simulink model "NewModel"  (R2020a)
settings: Solver=VariableStepAuto  StartTime=0.0  StopTime=500  RelTol=1e-3
values from neighbouring files (symbols this model uses):
  Ctr = 1.6    [ACC_DATA.m]
  F_aero = 1/(2*m_Follower)*Ro_A_Cd    (= 0.00026)    [ACC_DATA.m]
  F_grav = g*sin(theta)    [ACC_DATA.m]
  F_res = g*Cr*cos(theta)    [ACC_DATA.m]
  Kb = 0.08    [ACC_DATA.m]
  Kc = 1    [ACC_DATA.m]
  m_Follower = 1500    [ACC_DATA.m]
  r = 0.326    [ACC_DATA.m]
  Rf = 3.28    [ACC_DATA.m]
  Rtr = 1    [ACC_DATA.m]
  t_gap = 1.4    [ACC_DATA.m]    (also in Untitled.m)
  Tmax = 528.7 + 0.152*Ne - 0.0000217*Ne^2    (= 789.5)    [ACC_DATA.m]
  Ts = 0.1    [ACC_DATA.m]
  v0_lead = 20    [ACC_DATA.m]
  v_set = 40    [ACC_DATA.m]    (also in Untitled.m = 30)
  x0_ego = 10    [ACC_DATA.m]
  x0_lead = 500    [ACC_DATA.m]
undefined symbols (not defined in the file or in its folder): sigbuilder_block
libraries: simulink x2
settings Model: Creator=91968  LastModifiedBy=91968

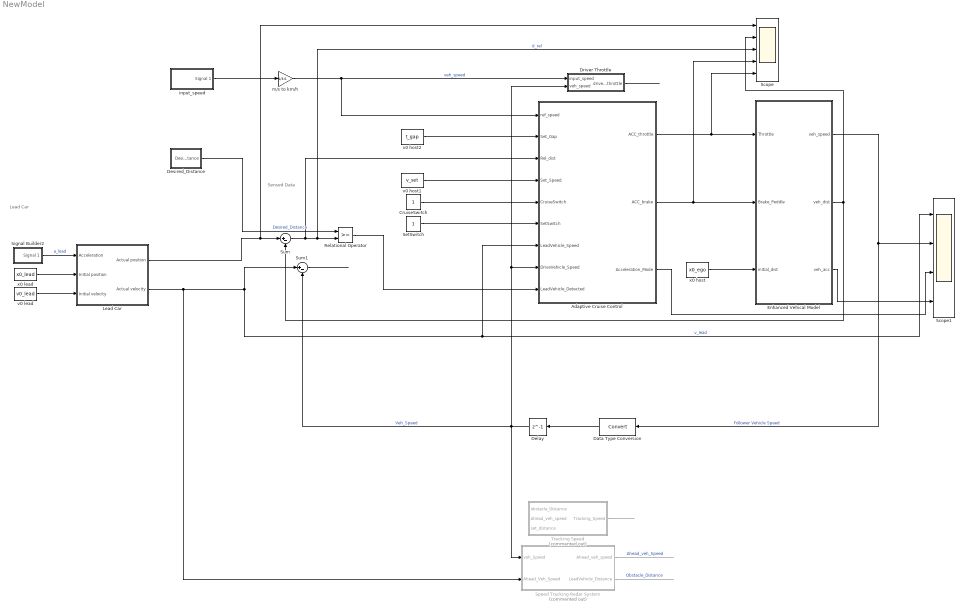
== system NewModel ==
  note: Lead Car
  note: Sensed Data
  Adaptive Cruise Control : Subsystem
  CruiseSwitch : Constant
  Data Type Conversion : DataTypeConversion
  Delay : Delay  DelayLength=1  InitialCondition=0
  Desired_Distance : Subsystem  mask{Desired_Distance=50.0}
      mask DialogControl DescGroupVar Prompt: Set Desired Distance
      mask Display: image('C:\Users\Talha Rao\Pictures\070558928_iconm (2).jpeg');
  Driver Throttle : Subsystem
  Enhanced Vehical Model : Subsystem
  Lead Car : Subsystem
  Relational Operator : RelationalOperator  OutDataTypeStr=boolean  RndMeth=Simplest
  Scope : Scope  NumInputPorts=5
  Scope1 : Scope  NumInputPorts=4
  SetSwitch : Constant
  Signal Builder2 : Subsystem  Tag=STV Subsys  LoadFcn=sigbuilder_block('load');  StartFcn=sigbuilder_block('start');  StopFcn=sigbuilder_block('stop');  ClipboardFcn=sigbuilder_block('clipboard');  mask(Sigbuilder block){tuvar=[0:10]}
      mask help: Simulink:masks:SigbuilderBlock_MD
      mask init:
      | if ~strcmp(get_param(bdroot(gcbh),'SimulationStatus'),'stopped') tuvar = sigbuilder_block('maskInit'); end
      settings: CopyFcn=sigbuilder_block('copy');  DeleteFcn=sigbuilder_block('delete');  ModelCloseFcn=sigbuilder_block('modelClose');  PreSaveFcn=sigbuilder_block('preSave');  PauseFcn=sigbuilder_block('pause');  ContinueFcn=sigbuilder_block('continue');  NameChangeFcn=sigbuilder_block('namechange');  OpenFcn=sigbuilder_block('open',[883.5 285.75 550.5 318.75 ]);  CloseFcn=sigbuilder_block('close');
      mask Display: plot(0, 0, 100, 100,[2, 2, 32, 32, 2], [68, 8, 8, 68, 68],[32, 2], [38, 38], [32, 19, 2],[53, 60, 44], [32, 17, 17, 2],[16, 16, 31, 31]);txt = getActiveGroup(gcbh);text(2, 100, txt,'verticalAlignment', 'top');
  Speed Tracking Redar System : Subsystem  Commented=on
  Sum : Sum  Inputs=|+-
  Sum1 : Sum  Inputs=|+-
  Tracking Speed : Subsystem  Commented=on
  input_speed : Subsystem  Tag=STV Subsys  LoadFcn=sigbuilder_block('load');  StartFcn=sigbuilder_block('start');  StopFcn=sigbuilder_block('stop');  ClipboardFcn=sigbuilder_block('clipboard');  mask(Sigbuilder block){tuvar=[0:10]}
      mask help: Simulink:masks:SigbuilderBlock_MD
      mask init:
      | if ~strcmp(get_param(bdroot(gcbh),'SimulationStatus'),'stopped') tuvar = sigbuilder_block('maskInit'); end
      settings: CopyFcn=sigbuilder_block('copy');  DeleteFcn=sigbuilder_block('delete');  ModelCloseFcn=sigbuilder_block('modelClose');  PreSaveFcn=sigbuilder_block('preSave');  PauseFcn=sigbuilder_block('pause');  ContinueFcn=sigbuilder_block('continue');  NameChangeFcn=sigbuilder_block('namechange');  OpenFcn=sigbuilder_block('open',[167.25 146.25 1152 549.75 ]);  CloseFcn=sigbuilder_block('close');
      mask Display: plot(0, 0, 100, 100,[2, 2, 32, 32, 2], [68, 8, 8, 68, 68],[32, 2], [38, 38], [32, 19, 2],[53, 60, 44], [32, 17, 17, 2],[16, 16, 31, 31]);txt = getActiveGroup(gcbh);text(2, 100, txt,'verticalAlignment', 'top');
  m/s to km/h : Gain  Gain=1/3.6
  v0 host1 : Constant  Value=v_set  SampleTime=Ts
  v0 host2 : Constant  Value=t_gap  SampleTime=Ts
  v0 lead : Constant  Value=v0_lead  SampleTime=Ts
  x0 host : Constant  Value=x0_ego  SampleTime=Ts
  x0 lead : Constant  Value=x0_lead  SampleTime=Ts
  wires:
  x0 lead/1 -> Lead Car/2(Initial position)
  v0 lead/1 -> Lead Car/3(Initial velocity)
  Signal Builder2/1(Signal 1) -> Lead Car/1(Acceleration)  "a_lead"
  Lead Car/1(Actual position) -> Scope/1, Sum/1
  Lead Car/2(Actual velocity) -> Speed Tracking Redar System/2(Ahead_Veh_Speed), Scope1/1, Adaptive Cruise Control/7(LeadVehicle_Speed), Sum1/1  "v_lead"
  Delay/1 -> Speed Tracking Redar System/1(veh_Speed), Sum1/2, Adaptive Cruise Control/8(DriveVehicle_Speed), Driver Throttle/2(veh_speed)  "Veh_Speed"
  Speed Tracking Redar System/2(LeadVehicle_Distance) -> ?  "Obstacle_Distance"
  Speed Tracking Redar System/1(Ahead_veh_speed) -> ?  "Ahead_veh_Speed"
  Desired_Distance/1(Desired_Distance) -> Relational Operator/1  "Desired_Distance"
  Enhanced Vehical Model/1(veh_speed) -> Scope1/2, Data Type Conversion/1  "Follower Vehicle Speed"
  Sum/1 -> Scope/3, Relational Operator/2, Adaptive Cruise Control/3(Rel_dist)  "d_rel"
  x0 host/1 -> Enhanced Vehical Model/3(initial_dist)
  Enhanced Vehical Model/2(veh_dist) -> Sum/2, Scope/2
  Data Type Conversion/1 -> Delay/1
  v0 host2/1 -> Adaptive Cruise Control/2(Set_Gap)
  v0 host1/1 -> Adaptive Cruise Control/4(Set_Speed)
  CruiseSwitch/1 -> Adaptive Cruise Control/5(CruiseSwitch)
  SetSwitch/1 -> Adaptive Cruise Control/6(SetSwitch)
  Relational Operator/1 -> Adaptive Cruise Control/9(LeadVehicle_Detected)
  input_speed/1(Signal 1) -> m/s to km/h/1
  Adaptive Cruise Control/1(ACC_throttle) -> Scope/5, Enhanced Vehical Model/1(Throttle)
  Adaptive Cruise Control/2(ACC_brake) -> Scope/4, Enhanced Vehical Model/2(Brake_Peddle)
  Tracking Speed/1(Tracking_Speed) -> ?
  Sum1/1 -> ?
  Driver Throttle/1(driver_throttle) -> ?
  Enhanced Vehical Model/3(veh_acc) -> Scope1/4
  Adaptive Cruise Control/3(Acceleration_Mode) -> Scope1/3
  m/s to km/h/1 -> Adaptive Cruise Control/1(ref_speed), Driver Throttle/1(input_speed)  "veh_speed"

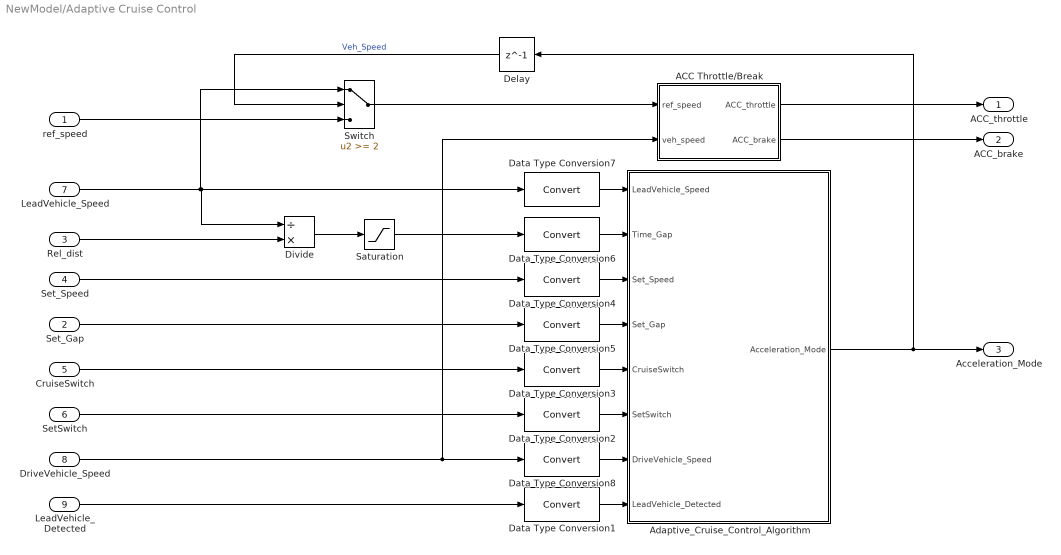
== system NewModel/Adaptive Cruise Control ==
  ref_speed : Inport
  Set_Gap : Inport  Port=2
  Rel_dist : Inport  Port=3
  Set_Speed : Inport  Port=4
  CruiseSwitch : Inport  Port=5
  SetSwitch : Inport  Port=6
  LeadVehicle_Speed : Inport  Port=7  OutMin=0  OutMax=255
  DriveVehicle_Speed : Inport  Port=8  OutMin=0  OutMax=255
  LeadVehicle_Detected : Inport  Port=9  OutMin=0  OutMax=1
  ACC Throttle/Break : Subsystem
  Adaptive_Cruise_Control_Algorithm : Subsystem
  Data Type Conversion{1..8} (8 alike) : DataTypeConversion
  Delay : Delay  DelayLength=1  InitialCondition=0
  Divide : Product  Inputs=/*
  Saturation : Saturate  UpperLimit=100  LowerLimit=0
  Switch : Switch  Threshold=2  SaturateOnIntegerOverflow=on  InputSameDT=on
  ACC_throttle : Outport
  ACC_brake : Outport  Port=2
  Acceleration_Mode : Outport  Port=3
  wires:
  Data Type Conversion7/1 -> Adaptive_Cruise_Control_Algorithm/1(LeadVehicle_Speed)
  Data Type Conversion4/1 -> Adaptive_Cruise_Control_Algorithm/3(Set_Speed)
  Data Type Conversion2/1 -> Adaptive_Cruise_Control_Algorithm/6(SetSwitch)
  Set_Speed/1 -> Data Type Conversion4/1
  Adaptive_Cruise_Control_Algorithm/1(Acceleration_Mode) -> Delay/1, Acceleration_Mode/1
  Data Type Conversion8/1 -> Adaptive_Cruise_Control_Algorithm/7(DriveVehicle_Speed)
  Data Type Conversion6/1 -> Adaptive_Cruise_Control_Algorithm/2(Time_Gap)
  Data Type Conversion3/1 -> Adaptive_Cruise_Control_Algorithm/5(CruiseSwitch)
  Data Type Conversion5/1 -> Adaptive_Cruise_Control_Algorithm/4(Set_Gap)
  Data Type Conversion1/1 -> Adaptive_Cruise_Control_Algorithm/8(LeadVehicle_Detected)
  Set_Gap/1 -> Data Type Conversion5/1
  Divide/1 -> Saturation/1
  ACC Throttle/Break/1(ACC_throttle) -> ACC_throttle/1
  CruiseSwitch/1 -> Data Type Conversion3/1
  ACC Throttle/Break/2(ACC_brake) -> ACC_brake/1
  LeadVehicle_Detected/1 -> Data Type Conversion1/1
  SetSwitch/1 -> Data Type Conversion2/1
  ref_speed/1 -> Switch/3
  DriveVehicle_Speed/1 -> ACC Throttle/Break/2(veh_speed), Data Type Conversion8/1
  LeadVehicle_Speed/1 -> Divide/1, Data Type Conversion7/1, Switch/1
  Rel_dist/1 -> Divide/2
  Saturation/1 -> Data Type Conversion6/1
  Switch/1 -> ACC Throttle/Break/1(ref_speed)
  Delay/1 -> Switch/2  "Veh_Speed"

== system NewModel/Desired_Distance ==
  Constant : Constant  Value=Desired_Distance
  Desired_Distance : Outport  VectorParamsAs1DForOutWhenUnconnected=off
  wires:
  Constant/1 -> Desired_Distance/1

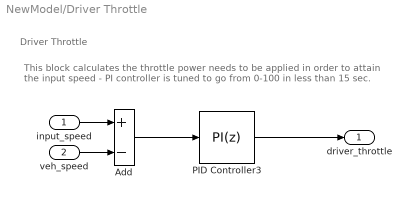
== system NewModel/Driver Throttle ==
  note: This block calculates the throttle power needs to be applied in order to attain the input speed
      | - PI controller is tuned to go from 0-100 in less than 15 sec.
  note: Driver Throttle
  input_speed : Inport
  veh_speed : Inport  Port=2
  Add : Sum  Inputs=+-
  PID Controller3 : simulink/Continuous/PID Controller  Controller=PI  Form=Parallel  TimeDomain=Discrete-time  UseExternalTs=off  SampleTime=0.02  IntegratorMethod=Trapezoidal  FilterMethod=Forward Euler  ControllerParametersSource=internal  P=5  I=0.5  D=0  UseFilter=on  N=100  TunerSelectOption=Transfer Function Based (PID Tuner App)  InitialConditionSource=internal  InitialConditionForIntegrator=0  InitialConditionForFilter=0  DifferentiatorICPrevScaledInput=0  ExternalReset=none  TrackingMode=off  Kt=1  LimitOutput=on  UpperSaturationLimit=100  LowerSaturationLimit=-100  LinearizeAsGain=on  AntiWindupMode=clamping  Kb=1  POutMin=[]  POutMax=[]  IOutMin=[]  IOutMax=[]  DOutMin=[]  DOutMax=[]  NOutMin=[]  NOutMax=[]  SumOutMin=[]  SumOutMax=[]  SaturationOutMin=[]  SaturationOutMax=[]  PParamMin=[]  PParamMax=[]  IParamMin=[]  IParamMax=[]  DParamMin=[]  DParamMax=[]  NParamMin=[]  NParamMax=[]  KbParamMin=[]  KbParamMax=[]  KtParamMin=[]  KtParamMax=[]  KbOutMin=[]  KbOutMax=[]  KtOutMin=[]  KtOutMax=[]  IntegratorOutMin=[]  IntegratorOutMax=[]  FilterOutMin=[]  FilterOutMax=[]  SumI1OutMin=[]  SumI1OutMax=[]  SumI2OutMin=[]  SumI2OutMax=[]  SumI3OutMin=[]  SumI3OutMax=[]  SumI4OutMin=[]  SumI4OutMax=[]  SumDOutMin=[]  SumDOutMax=[]  DifferentiatorOutMin=[]  DifferentiatorOutMax=[]  FilterDiffOutCoefMin=[]  FilterDiffOutCoefMax=[]  ReciprocalOutMin=[]  ReciprocalOutMax=[]  SumDenOutMin=[]  SumDenOutMax=[]  SumNumOutMin=[]  SumNumOutMax=[]  DivideOutMin=[]  DivideOutMax=[]  UdiffTsProdOutMin=[]  UdiffTsProdOutMax=[]  NTsProdOutMin=[]  NTsProdOutMax=[]  UintegralTsProdOutMin=[]  UintegralTsProdOutMax=[]  UngainTsProdOutMin=[]  UngainTsProdOutMax=[]  IntegratorContinuousStateAttributes=''  IntegratorStateMustResolveToSignalObject=off  IntegratorRTWStateStorageClass=Auto  FilterContinuousStateAttributes=''  FilterStateMustResolveToSignalObject=off  FilterRTWStateStorageClass=Auto  ParallelPVariant=InternalParameters  IdealPVariant=Disabled  IVariant=InternalParameters  DVariant=Disabled  IntegratorVariant=Discrete  SatVariant=Enabled  AWVariant=DiscClampingParallel  PCopyVariant=Disabled  TRVariant=Disabled  FdbkBlocksVariant=Feedback  IdealPFdbkVariant=Passthrough  SatFdbkVariant=Passthrough  DerivativeFilterVariant=Disabled  NVariant=Disabled  NCopyVariant=Disabled_SignalSpec  FilterICVariant=Disabled  IntegratorICVariant=InternalICs  ExternalResetVariant=Disabled  TRSumVariant=Passthrough  SumFdbkVariant=Enabled  SumVariant=Sum_PI  TsampFilterVariant=InternalTs  TsampNgainVariant=Passthrough  TsampIntegralVariant=Passthrough
  driver_throttle : Outport  VectorParamsAs1DForOutWhenUnconnected=off
  wires:
  input_speed/1 -> Add/1
  veh_speed/1 -> Add/2
  PID Controller3/1 -> driver_throttle/1
  Add/1 -> PID Controller3/1

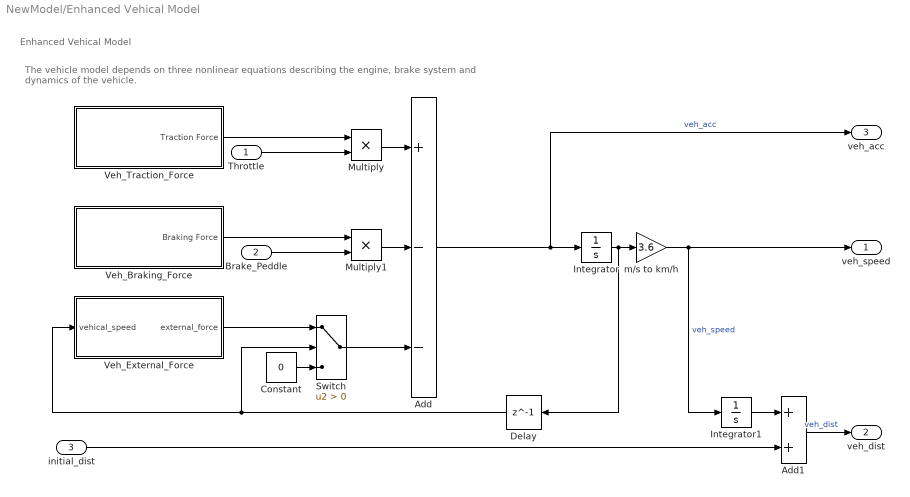
== system NewModel/Enhanced Vehical Model ==
  note: The vehicle model depends on three nonlinear equations describing the engine, brake system and dynamics of the vehicle.
  note: Enhanced Vehical Model
  Throttle : Inport
  Brake_Peddle : Inport  Port=2
  initial_dist : Inport  Port=3
  Add : Sum  Inputs=+--
  Add1 : Sum
  Constant : Constant  Value=0
  Delay : Delay  DelayLength=1  InitialCondition=0
  Integrator : Integrator
  Integrator1 : Integrator
  Multiply : Product
  Multiply1 : Product
  Switch : Switch  Criteria=u2 > Threshold  SaturateOnIntegerOverflow=on  InputSameDT=on
  Veh_Braking_Force : Subsystem
  Veh_External_Force : Subsystem
  Veh_Traction_Force : Subsystem
  m/s to km/h : Gain  Gain=3.6
  veh_speed : Outport  VectorParamsAs1DForOutWhenUnconnected=off
  veh_dist : Outport  Port=2  VectorParamsAs1DForOutWhenUnconnected=off
  veh_acc : Outport  Port=3  VectorParamsAs1DForOutWhenUnconnected=off
  wires:
  Switch/1 -> Add/3
  Brake_Peddle/1 -> Multiply1/2
  Veh_Braking_Force/1("Braking Force ") -> Multiply1/1
  Multiply1/1 -> Add/2
  Multiply/1 -> Add/1
  Veh_Traction_Force/1(Traction Force) -> Multiply/1
  Integrator/1 -> Delay/1, m/s to km/h/1
  m/s to km/h/1 -> Integrator1/1, veh_speed/1  "veh_speed"
  Integrator1/1 -> Add1/1
  Add1/1 -> veh_dist/1  "veh_dist"
  initial_dist/1 -> Add1/2
  Delay/1 -> Switch/2, Veh_External_Force/1(vehical_speed)
  Veh_External_Force/1(external_force) -> Switch/1
  Constant/1 -> Switch/3
  Add/1 -> veh_acc/1, Integrator/1  "veh_acc"
  Throttle/1 -> Multiply/2

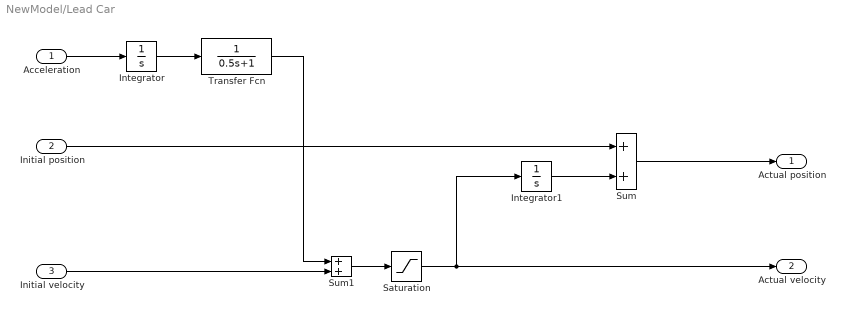
== system NewModel/Lead Car ==
  Acceleration : Inport
  Initial position : Inport  Port=2
  Initial velocity : Inport  Port=3
  Integrator : Integrator
  Integrator1 : Integrator
  Saturation : Saturate  UpperLimit=50  LowerLimit=0
  Sum : Sum
  Sum1 : Sum
  Transfer Fcn : TransferFcn  Denominator=[0.5 1]
  Actual position : Outport  VectorParamsAs1DForOutWhenUnconnected=off
  Actual velocity : Outport  Port=2  VectorParamsAs1DForOutWhenUnconnected=off
  wires:
  Transfer Fcn/1 -> Sum1/1
  Initial velocity/1 -> Sum1/2
  Sum/1 -> Actual position/1
  Integrator/1 -> Transfer Fcn/1
  Sum1/1 -> Saturation/1
  Acceleration/1 -> Integrator/1
  Initial position/1 -> Sum/1
  Integrator1/1 -> Sum/2
  Saturation/1 -> Integrator1/1, Actual velocity/1

== system NewModel/Signal Builder2 ==
  Demux : Demux  Tag=STV Demux  Outputs=1
      settings: DisplayOption=none
  FromWs : FromWorkspace  Tag=STV FromWs  VariableName=tuvar
      SigBuilderData=|
      | common.afterFinalStr = 'Extrapolate'
      | common.sampleTime = 0
      | dataSet.timeRange = [0 500]
      | dataSet.name = 'Group 1'
      | sbobj.Groups.Name = 'Group 1'
      | sbobj.Groups.Signals.Name = 'Signal 1'
      | sbobj.Groups.Signals.XData = [0 20 30 40 60 80 100 150 200 250 300 350 400 451 500]
      | sbobj.Groups.Signals.YData = [0.5 1 1.5 1.5 0.75 -1 -1.8 0 -0.5 -3 0.5 -0.25 -1 -1 -1.5]
      | sbobj.Groups.TimeRange = [0 500]
  Signal 1 : Outport  Tag=STV Outport
  wires:
  Demux/1 -> Signal 1/1
  FromWs/1 -> Demux/1

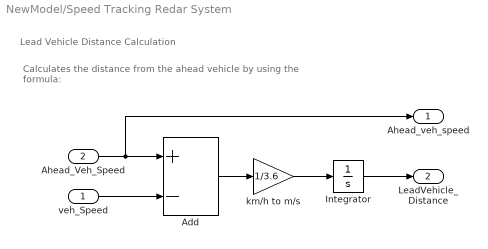
== system NewModel/Speed Tracking Redar System ==
  note: Calculates the distance from the ahead vehicle by using the formula:
  note: Lead Vehicle Distance Calculation
  veh_Speed : Inport
  Ahead_Veh_Speed : Inport  Port=2
  Add : Sum  Inputs=+-
  Integrator : Integrator  InitialCondition=100
  km/h to m/s : Gain  Gain=1/3.6
  Ahead_veh_speed : Outport  VectorParamsAs1DForOutWhenUnconnected=off
  LeadVehicle_Distance : Outport  Port=2  VectorParamsAs1DForOutWhenUnconnected=off
  wires:
  Ahead_Veh_Speed/1 -> Ahead_veh_speed/1, Add/1
  veh_Speed/1 -> Add/2
  Add/1 -> km/h to m/s/1
  km/h to m/s/1 -> Integrator/1
  Integrator/1 -> LeadVehicle_Distance/1

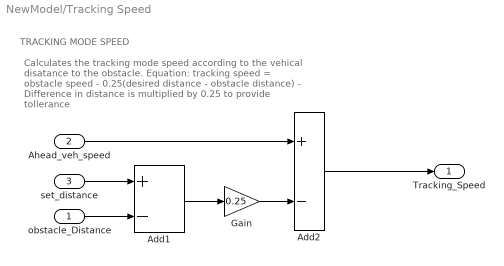
== system NewModel/Tracking Speed ==
  note: Calculates the tracking mode speed according to the vehical disatance
      | to the obstacle.
      | Equation:
      |
      | tracking speed = obstacle speed - 0.25(desired distance - obstacle distance)
      |
      | - Difference in distance is multiplied by 0.25 to provide tollerance
  note: TRACKING MODE SPEED
  obstacle_Distance : Inport
  Ahead_veh_speed : Inport  Port=2
  set_distance : Inport  Port=3
  Add1 : Sum  Inputs=+-
  Add2 : Sum  Inputs=+-
  Gain : Gain  Gain=0.25
  Tracking_Speed : Outport  VectorParamsAs1DForOutWhenUnconnected=off
  wires:
  Add1/1 -> Gain/1
  Gain/1 -> Add2/2
  Ahead_veh_speed/1 -> Add2/1
  Add2/1 -> Tracking_Speed/1
  set_distance/1 -> Add1/1
  obstacle_Distance/1 -> Add1/2

== system NewModel/input_speed ==
  Demux : Demux  Tag=STV Demux  Outputs=1
      settings: DisplayOption=none
  FromWs : FromWorkspace  Tag=STV FromWs  VariableName=tuvar
      SigBuilderData=|
      | common.afterFinalStr = 'Extrapolate'
      | common.sampleTime = 0
      | dataSet.timeRange = [0 500]
      | dataSet.name = 'Group 1'
      | sbobj.Groups.Name = 'Group 1'
      | sbobj.Groups.Signals.Name = 'Signal 1'
      | sbobj.Groups.Signals.XData = [0 20 30 40 60 80 100 150 200 250 300 350 400 451 500]
      | sbobj.Groups.Signals.YData = [0.5 15.5 25.5 40.5 40.5 75.5 75.5 70.5 60.5 60 90 90 60 45 40]
      | sbobj.Groups.TimeRange = [0 500]
  Signal 1 : Outport  Tag=STV Outport
  wires:
  Demux/1 -> Signal 1/1
  FromWs/1 -> Demux/1

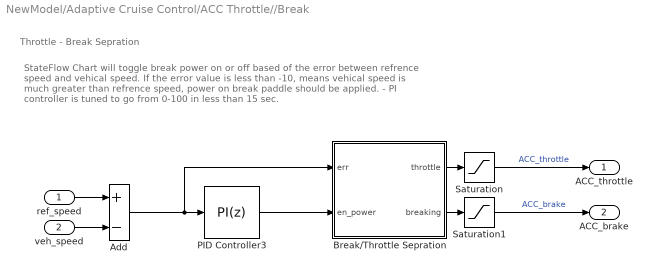
== system NewModel/Adaptive Cruise Control/ACC Throttle//Break ==
  note: StateFlow Chart will toggle break power on or off based of the error between refrence speed and
      | vehical speed. If the error value is less than -10, means vehical speed is much greater than refrence
      | speed, power on break paddle should be applied.
      |
      | - PI controller is tuned to go from 0-100 in less than 15 sec.
  note: Throttle - Break Sepration
  ref_speed : Inport
  veh_speed : Inport  Port=2
  Add : Sum  Inputs=+-
  Break/Throttle Sepration : Stateflow chart  TreatAsAtomicUnit=on
  PID Controller3 : simulink/Continuous/PID Controller  Controller=PI  Form=Parallel  TimeDomain=Discrete-time  UseExternalTs=off  SampleTime=0.02  IntegratorMethod=Trapezoidal  FilterMethod=Forward Euler  ControllerParametersSource=internal  P=2  I=5  D=0  UseFilter=on  N=100  TunerSelectOption=Transfer Function Based (PID Tuner App)  InitialConditionSource=internal  InitialConditionForIntegrator=0  InitialConditionForFilter=0  DifferentiatorICPrevScaledInput=0  ExternalReset=none  TrackingMode=off  Kt=1  LimitOutput=on  UpperSaturationLimit=100  LowerSaturationLimit=-100  LinearizeAsGain=on  AntiWindupMode=clamping  Kb=1  POutMin=[]  POutMax=[]  IOutMin=[]  IOutMax=[]  DOutMin=[]  DOutMax=[]  NOutMin=[]  NOutMax=[]  SumOutMin=[]  SumOutMax=[]  SaturationOutMin=[]  SaturationOutMax=[]  PParamMin=[]  PParamMax=[]  IParamMin=[]  IParamMax=[]  DParamMin=[]  DParamMax=[]  NParamMin=[]  NParamMax=[]  KbParamMin=[]  KbParamMax=[]  KtParamMin=[]  KtParamMax=[]  KbOutMin=[]  KbOutMax=[]  KtOutMin=[]  KtOutMax=[]  IntegratorOutMin=[]  IntegratorOutMax=[]  FilterOutMin=[]  FilterOutMax=[]  SumI1OutMin=[]  SumI1OutMax=[]  SumI2OutMin=[]  SumI2OutMax=[]  SumI3OutMin=[]  SumI3OutMax=[]  SumI4OutMin=[]  SumI4OutMax=[]  SumDOutMin=[]  SumDOutMax=[]  DifferentiatorOutMin=[]  DifferentiatorOutMax=[]  FilterDiffOutCoefMin=[]  FilterDiffOutCoefMax=[]  ReciprocalOutMin=[]  ReciprocalOutMax=[]  SumDenOutMin=[]  SumDenOutMax=[]  SumNumOutMin=[]  SumNumOutMax=[]  DivideOutMin=[]  DivideOutMax=[]  UdiffTsProdOutMin=[]  UdiffTsProdOutMax=[]  NTsProdOutMin=[]  NTsProdOutMax=[]  UintegralTsProdOutMin=[]  UintegralTsProdOutMax=[]  UngainTsProdOutMin=[]  UngainTsProdOutMax=[]  IntegratorContinuousStateAttributes=''  IntegratorStateMustResolveToSignalObject=off  IntegratorRTWStateStorageClass=Auto  FilterContinuousStateAttributes=''  FilterStateMustResolveToSignalObject=off  FilterRTWStateStorageClass=Auto  ParallelPVariant=InternalParameters  IdealPVariant=Disabled  IVariant=InternalParameters  DVariant=Disabled  IntegratorVariant=Discrete  SatVariant=Enabled  AWVariant=DiscClampingParallel  PCopyVariant=Disabled  TRVariant=Disabled  FdbkBlocksVariant=Feedback  IdealPFdbkVariant=Passthrough  SatFdbkVariant=Passthrough  DerivativeFilterVariant=Disabled  NVariant=Disabled  NCopyVariant=Disabled_SignalSpec  FilterICVariant=Disabled  IntegratorICVariant=InternalICs  ExternalResetVariant=Disabled  TRSumVariant=Passthrough  SumFdbkVariant=Enabled  SumVariant=Sum_PI  TsampFilterVariant=InternalTs  TsampNgainVariant=Passthrough  TsampIntegralVariant=Passthrough
  Saturation : Saturate  UpperLimit=50  LowerLimit=0
  Saturation1 : Saturate  UpperLimit=20  LowerLimit=0
  ACC_throttle : Outport  VectorParamsAs1DForOutWhenUnconnected=off
  ACC_brake : Outport  Port=2  VectorParamsAs1DForOutWhenUnconnected=off
  wires:
  ref_speed/1 -> Add/1
  veh_speed/1 -> Add/2
  Break/Throttle Sepration/1(throttle) -> Saturation/1
  Break/Throttle Sepration/2(breaking) -> Saturation1/1
  PID Controller3/1 -> Break/Throttle Sepration/2(en_power)
  Add/1 -> Break/Throttle Sepration/1(err), PID Controller3/1
  Saturation/1 -> ACC_throttle/1  "ACC_throttle"
  Saturation1/1 -> ACC_brake/1  "ACC_brake"

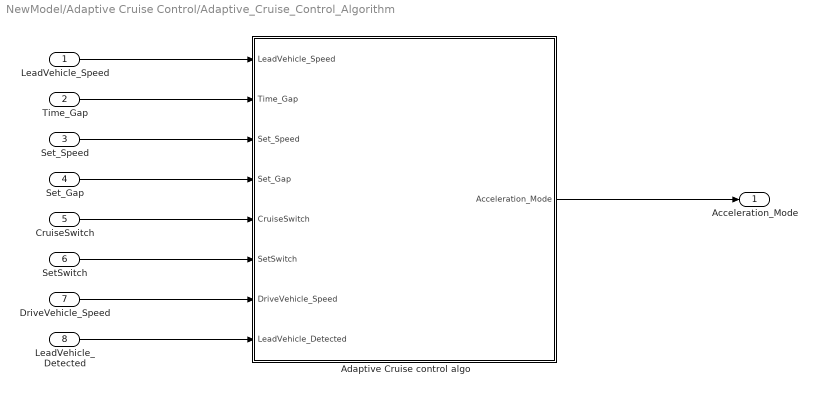
== system NewModel/Adaptive Cruise Control/Adaptive_Cruise_Control_Algorithm ==
  LeadVehicle_Speed : Inport  OutMin=0  OutMax=255
  Time_Gap : Inport  Port=2
  Set_Speed : Inport  Port=3
  Set_Gap : Inport  Port=4
  CruiseSwitch : Inport  Port=5
  SetSwitch : Inport  Port=6
  DriveVehicle_Speed : Inport  Port=7  OutMin=0  OutMax=255
  LeadVehicle_Detected : Inport  Port=8  OutMin=0  OutMax=255
  Adaptive Cruise control algo : Stateflow chart  RequirementInfo={} %GIDa_57645b32_15f0_49df_b2ac_141007f7ec66  TreatAsAtomicUnit=on
  Acceleration_Mode : Outport  OutMin=0  OutMax=255
  wires:
  LeadVehicle_Speed/1 -> Adaptive Cruise control algo/1(LeadVehicle_Speed)
  Set_Gap/1 -> Adaptive Cruise control algo/4(Set_Gap)
  Set_Speed/1 -> Adaptive Cruise control algo/3(Set_Speed)
  Time_Gap/1 -> Adaptive Cruise control algo/2(Time_Gap)
  LeadVehicle_Detected/1 -> Adaptive Cruise control algo/8(LeadVehicle_Detected)
  DriveVehicle_Speed/1 -> Adaptive Cruise control algo/7(DriveVehicle_Speed)
  SetSwitch/1 -> Adaptive Cruise control algo/6(SetSwitch)
  CruiseSwitch/1 -> Adaptive Cruise control algo/5(CruiseSwitch)
  Adaptive Cruise control algo/1(Acceleration_Mode) -> Acceleration_Mode/1

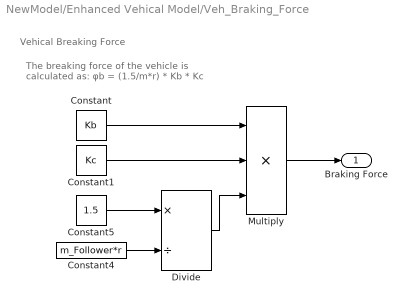
== system NewModel/Enhanced Vehical Model/Veh_Braking_Force ==
  note: Vehical Breaking Force
  note: The breaking force of the vehicle is calculated as:
      | φb = (1.5/m*r) * Kb * Kc
  Constant : Constant  Value=Kb
  Constant1 : Constant  Value=Kc
  Constant4 : Constant  Value=m_Follower*r
  Constant5 : Constant  Value=1.5
  Divide : Product  Inputs=*/
  Multiply : Product  Inputs=3
  "Braking Force " : Outport  VectorParamsAs1DForOutWhenUnconnected=off
  wires:
  Multiply/1 -> "Braking Force "/1
  Constant4/1 -> Divide/2
  Constant1/1 -> Multiply/2
  Constant/1 -> Multiply/1
  Constant5/1 -> Divide/1
  Divide/1 -> Multiply/3

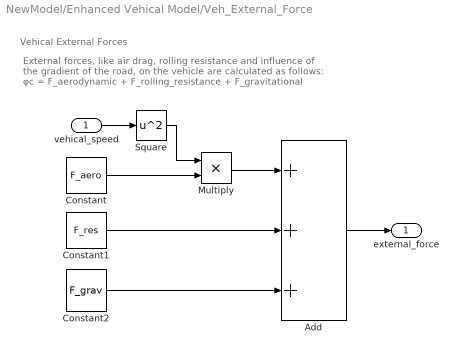
== system NewModel/Enhanced Vehical Model/Veh_External_Force ==
  note: External forces, like air drag, rolling resistance and
      | influence of the gradient of the road, on the vehicle are calculated as follows:
      |
      | φc = F_aerodynamic + F_rolling_resistance + F_gravitational
  note: Vehical External Forces
  vehical_speed : Inport
  Add : Sum  Inputs=+++
  Constant : Constant  Value=F_aero
  Constant1 : Constant  Value=F_res
  Constant2 : Constant  Value=F_grav
  Multiply : Product
  Square : Math  Operator=square  SignedPower=on  SaturateOnIntegerOverflow=on
  external_force : Outport  VectorParamsAs1DForOutWhenUnconnected=off
  wires:
  Add/1 -> external_force/1
  Constant1/1 -> Add/2
  Constant2/1 -> Add/3
  Constant/1 -> Multiply/2
  vehical_speed/1 -> Square/1
  Square/1 -> Multiply/1
  Multiply/1 -> Add/1

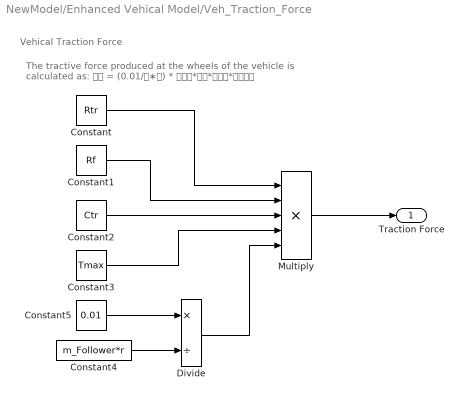
== system NewModel/Enhanced Vehical Model/Veh_Traction_Force ==
  note: The tractive force produced at the wheels of the vehicle is calculated as:
      | 𝜑𝑡 = (0.01/𝑚∗𝑟) * 𝑅𝑡𝑟*𝑅𝑓*𝐶𝑡𝑟*𝑇𝑚𝑎𝑥
  note: Vehical Traction Force
  Constant : Constant  Value=Rtr
  Constant1 : Constant  Value=Rf
  Constant2 : Constant  Value=Ctr
  Constant3 : Constant  Value=Tmax
  Constant4 : Constant  Value=m_Follower*r
  Constant5 : Constant  Value=0.01
  Divide : Product  Inputs=*/
  Multiply : Product  Inputs=5
  Traction Force : Outport  VectorParamsAs1DForOutWhenUnconnected=off
  wires:
  Constant/1 -> Multiply/1
  Constant4/1 -> Divide/2
  Constant1/1 -> Multiply/2
  Constant5/1 -> Divide/1
  Constant3/1 -> Multiply/4
  Divide/1 -> Multiply/5
  Constant2/1 -> Multiply/3
  Multiply/1 -> Traction Force/1

== stateflow chart NewModel/Adaptive Cruise Control/ACC Throttle//Break/Break//Throttle Sepration ==
  note: Break/Throttle Separation
  note: State
      | Description
      | Condition
      | Next State
      |
      | OPEN_THROTTLE
      | Apply power on throttle when error is >= -10
      | err >= -10
      | APPLY_BREAK
      |
      | APPLY_BREAK
      | Apply power on break when error is < -10
      | err < -10
      | OPEN_THROTTLE
  state OPEN_THROTTLE
    en: breaking = 0;
    during: throttle = en_power;
  state APPLY_BREAK
    during: breaking = en_power;
    en:throttle = 0;
  (default) -> OPEN_THROTTLE
  OPEN_THROTTLE -> APPLY_BREAK : [err<-5]
  APPLY_BREAK -> OPEN_THROTTLE : [err >= 0]
  data: throttle output; breaking output; err input; en_power input

== stateflow chart NewModel/Adaptive Cruise Control/Adaptive_Cruise_Control_Algorithm/Adaptive Cruise control algo ==
  state ACC_STANDBY_MODE
    entry:
    Acceleration_Mode = 1;
  state ACC_OFF_MODE
    entry:
    Acceleration_Mode = 0;
  state ACC_ON_MODE
    state LeadVehicle_Not_Detected_Resume
      entry:
      Acceleration_Mode= 1;
    state LeadVehicle_Detected_Resume
      entry:
      Acceleration_Mode= 3;
    state LeadVehicle_Detected_Follow
      entry:
      Acceleration_Mode= 2;
    state LeadVehicle_Not_Detected
      entry:
      Acceleration_Mode= 1;
    state LeadVehicle_Speed_equal_Set_Speed
      entry:
      Acceleration_Mode= 4;
    state LeadVehicle_Speed_lessthan_Set_Speed
      entry:
      Acceleration_Mode= 5;
    (default) -> LeadVehicle_Detected_Follow
    LeadVehicle_Detected_Resume -> LeadVehicle_Not_Detected_Resume [order 1] : [LeadVehicle_Detected ==0]
    LeadVehicle_Detected_Follow -> LeadVehicle_Detected_Resume [order 3] : [(DriveVehicle_Speed==Set_Speed) ...
        | && (LeadVehicle_Speed >= Set_Speed)...
        |  && (Time_Gap>=Set_Gap)]
    LeadVehicle_Speed_lessthan_Set_Speed -> LeadVehicle_Not_Detected_Resume [order 2] : [(LeadVehicle_Detected==0) ...
        | || (DriveVehicle_Speed <= Set_Speed)]
    LeadVehicle_Detected_Resume -> LeadVehicle_Speed_lessthan_Set_Speed [order 2] : [(DriveVehicle_Speed< Set_Speed) ...
        | && (LeadVehicle_Speed > DriveVehicle_Speed)...
        | || (Time_Gap >= Set_Gap)]
    LeadVehicle_Speed_lessthan_Set_Speed -> LeadVehicle_Detected_Resume [order 1] : [(DriveVehicle_Speed< Set_Speed) ...
        | && (LeadVehicle_Speed > DriveVehicle_Speed)...
        | && (Time_Gap >= Set_Gap)]
    LeadVehicle_Detected_Follow -> LeadVehicle_Not_Detected [order 2] : [LeadVehicle_Detected ==0]
    LeadVehicle_Not_Detected -> LeadVehicle_Detected_Follow [order 1] : [(LeadVehicle_Detected==1) && ...
        | (DriveVehicle_Speed == Set_Speed) && ...
        |  (LeadVehicle_Speed >= Set_Speed) &&...
        |  (Time_Gap>=Set_Gap)]
    LeadVehicle_Detected_Follow -> LeadVehicle_Speed_equal_Set_Speed [order 1] : [(LeadVehicle_Detected==1) ...
        | && (LeadVehicle_Speed < Set_Speed)...
        |  || (Time_Gap<Set_Gap)]
    LeadVehicle_Speed_equal_Set_Speed -> LeadVehicle_Not_Detected [order 1] : [(LeadVehicle_Detected==0) && ...
        | (DriveVehicle_Speed == Set_Speed)]
    LeadVehicle_Not_Detected -> LeadVehicle_Speed_equal_Set_Speed [order 2] : [(LeadVehicle_Detected==1) ...
        | && (LeadVehicle_Speed < Set_Speed)...
        |  || (Time_Gap<Set_Gap)]
    LeadVehicle_Speed_lessthan_Set_Speed -> LeadVehicle_Speed_equal_Set_Speed [order 3] : [(LeadVehicle_Speed< Set_Speed) ...
        | && (LeadVehicle_Speed < DriveVehicle_Speed)...
        | || (Time_Gap == 0.75*Set_Gap)]
    LeadVehicle_Speed_equal_Set_Speed -> LeadVehicle_Speed_lessthan_Set_Speed [order 2] : [(LeadVehicle_Speed*1.25 >= DriveVehicle_Speed) ...
        | && (LeadVehicle_Speed*0.75 <= DriveVehicle_Speed)...
        | && (DriveVehicle_Speed < Set_Speed) && (Time_Gap <=1.25*Set_Gap)...
        | && (Time_Gap >= 0.75*Set_Gap)]
  note: State
      | Description
      | Condition
      | Next State
      |
      | IDLE_STATE
      | Set cc refrence speed & set_speed equal to input speed
      | default || ACC_OFF
      | SPEED_TRACKING
      |
      | SPEED_TRACKING
      | Follow the set speed chosen by the driver
      | ACC_ON event occured && obstacle_distance < set_distance
      | DISTANCE_TRACKING / IDLE_STATE
      |
      | DISTANCE_TRACKING
      | Follow the tracking speed to keep the min distance maintained
      | obstacle_distance > set_distance...
      | && after(60,sec)
      | SPEED_TRACKING
  (default) -> ACC_OFF_MODE
  ACC_OFF_MODE -> ACC_STANDBY_MODE : [CruiseSwitch == 1]
  ACC_STANDBY_MODE -> ACC_OFF_MODE [order 1] : [CruiseSwitch==0]
  ACC_ON_MODE -> ACC_STANDBY_MODE : [SetSwitch ==0]
  ACC_STANDBY_MODE -> ACC_ON_MODE [order 2] : [SetSwitch ==1]
  data: LeadVehicle_Speed input; Time_Gap input; Set_Speed input; Set_Gap input; CruiseSwitch input [0..1]; SetSwitch input [0..1]; DriveVehicle_Speed input; LeadVehicle_Detected input; Acceleration_Mode output
